simulink subsystem "cvrs_ventricle_volume_systole"  (R2019b)
settings: Solver=VariableStepAuto  StartTime=0.0  StopTime=10.0  RelTol=1e-3
settings Model: Creator=RH  LastModifiedBy=RH

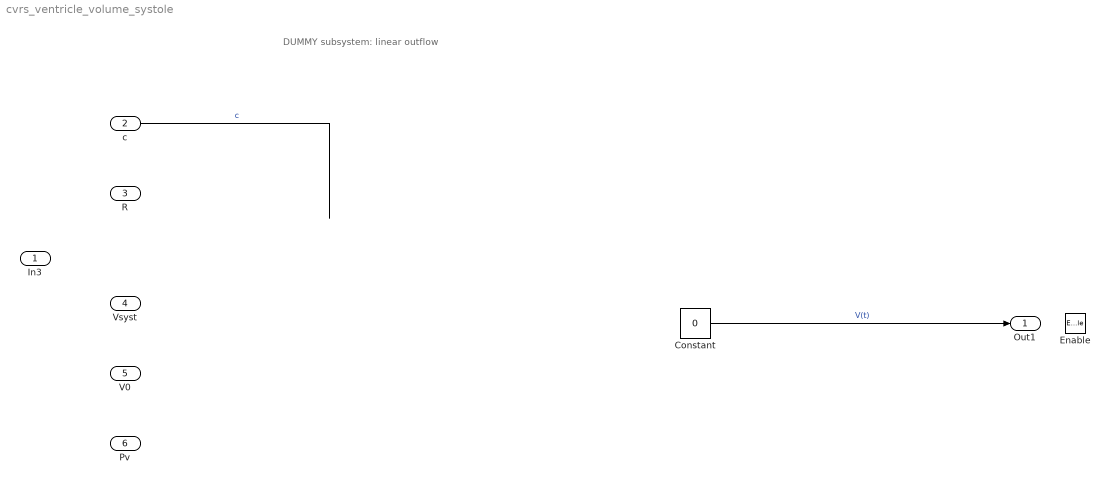
== system cvrs_ventricle_volume_systole ==
  note: DUMMY subsystem: linear outflow
  In3 : Inport
  c : Inport  Port=2
  R : Inport  Port=3
  Vsyst : Inport  Port=4
  V0 : Inport  Port=5
  Pv : Inport  Port=6
  Enable : EnablePort
  Constant : Constant  Value=0
  Out1 : Outport
  wires:
  c/1 -> ?  "c"
  Constant/1 -> Out1/1  "V(t)"
